simulink model "abl_M1_proposed"  (R2023b)
settings: Solver=ode45  StartTime=0.0  StopTime=80  MaxStep=1e-3  RelTol=5e-5
model workspace (MAT data in the model file):
  gpsid1 : Simulink.Signal (value not decoded)
  gpsid2 : Simulink.Signal (value not decoded)
  gpsid3 : Simulink.Signal (value not decoded)
  kkk1 : Simulink.Signal (value not decoded)
  kkk2 : Simulink.Signal (value not decoded)
  kkk3 : Simulink.Signal (value not decoded)
  psid = 0.5
undefined symbols (not defined in the file): A_raw1, A_raw2, beta1, beta2, p00, p_d_10, p_d_20, p_d_30, p_d_40, p_d_50, p_d_60, p_hat_p10, p_hat_p20, p_hat_p30, p_hat_p40, p_hat_p50, p_hat_p60, p_hat_v10, p_hat_v20, p_hat_v30, p_hat_v40, p_hat_v50, p_hat_v60, p_off_set1, p_off_set2, v00
(part 4 of 4)

== matlab function abl_M1_proposed/MATLAB Function1 ==
  settings: updateMethod=DISCRETE
  data: t input; dp_hat_i output; p0 input; v0 input; p_hat_all input; v_hat_all input; p_d_all input; id input; A_row input; beta input; p_offset input; dv_hat_i output; dp_d_i output
function [dp_hat_i, dv_hat_i, dp_d_i] = Follower_Model(t, p0, v0, p_hat_all, v_hat_all, p_d_all, id, A_row, beta, p_offset)
    % 输入说明:
    % t: 仿真时间 (Clock)
    % p0, v0: 领航者真实状态 (仅在beta_i > 0时起作用)
    % p_hat_all, v_hat_all, p_d_all: 所有跟随者的状态矩阵 (外部合并后传入)
    % id: 当前智能体编号
    % A_row: 当前智能体对其他人的邻接权重 (用于检测网络拓扑变化)
    % beta_i: 当前智能体是否能直接观测到领航者 (1或0)
    % p_offset: 期望与目标的相对编队位置偏置 (2x1 向量)

    % --- 仿真参数设定 ---
    kp_l = 0.5; 
    phi_p = 2.0; 
    Ta = 5.0;         % 规定观测器收敛时间
    Omega_bar = 4; 
    k1 = 0.1; 
    lambda = 1.0; 
    Tp = 10.0;      % 规定围住控制形成的时间
    d_avoid = 10;    % 避碰距离 d
    mu = 20;         % 避碰范围上限 mu

    % === 自动重启机制核心逻辑 ===
    % 使用 persistent 变量存储上一时刻的拓扑和最近一次的切换时间 tk
    persistent tk A_row_prev;
    
    if isempty(tk)
        tk = 0;
        A_row_prev = A_row;
    end
    
    % 检测到邻接权重矩阵发生改变，说明有智能体加入/退出，更新重启时刻 tk
    if any(A_row ~= A_row_prev)
        tk = t;
        A_row_prev = A_row;
    end
    
    % 计算自上次拓扑切换以来经过的“局部时间”
    t_local = t - tk; 
    % ===========================

    p_hat_i = p_hat_all(2*(id-1)+1:2*id);
    v_hat_i = v_hat_all(2*(id-1)+1:2*id);
    p_d_i = p_d_all(2*(id-1)+1:2*id);

    %% ---------------- A. 移动目标规定时间观测器 ----------------
    sum_p = zeros(size(p_hat_i));
    sum_v = zeros(size(v_hat_i));
    % 这里的循环处理完美契合“无标签”特性：不管是谁，只要 A_row(j)>0 就计算
    for j = 1:size(beta, 1)
        if A_row(id,j) > 0 && j ~= id
            sum_p = sum_p + A_row(id,j) * (p_hat_i - p_hat_all(2*(j-1)+1:2*j));
            sum_v = sum_v + A_row(id,j) * (v_hat_i - v_hat_all(2*(j-1)+1:2*j));
        end
    end
    
    eta_ip = sum_p + beta(id) * (p_hat_i - p0);
    eta_iv = sum_v + beta(id) * (v_hat_i - v0);

    % 观测器时变增益 kp (基于局部时间 t_local 重启)
    % 引入 -0.01 防止时间刚好等于 Ta 时分母为 0
    if t_local < Ta - 0.001 
        kp = kp_l + 1/(2*phi_p) + 2/(Ta - t_local);
    else
        kp = kp_l + 1/(2*phi_p);
    end

    sig_eta_iv = sign(eta_iv); 
    dp_hat_i = v_hat_i - kp * eta_ip;
    dv_hat_i = -kp * eta_iv - Omega_bar * sig_eta_iv;

    %% ---------------- B. 无标签目标围捕导航层 ----------------
    % 导航层时变增益 k (基于局部时间 t_local 重启)
    if t_local < Tp - 0.2
        k_gain = k1 + 0.01 + lambda/(Tp - t_local);
    else
        k_gain = k1 + 0.01;
    end

    p_tilde_d_i = p_d_i - p_hat_i - 0*p_offset(:,id); 
    m_gain = 100;
    sum_avoid = zeros(size(p_d_i));
    for j = 1:size(beta, 1)
        if A_row(id,j) > 0 && j ~= id
            p_d_ij = p_d_i - p_d_all(2*(j-1)+1:2*j);
            norm_p = norm(p_d_ij);
            
            if norm_p > d_avoid && norm_p <= mu
                alpha_val = 1/(norm_p - d_avoid) - 1/(mu - d_avoid);
            else
                alpha_val = 0; % 超出感知范围，或者发生了不可逆穿透，斥力置0防崩溃
            end
            
            if norm_p > 0
                % + 号表示顺着 p_d_ij 的方向把自己推开
                sum_avoid = sum_avoid + m_gain * alpha_val * (p_d_ij / norm_p);
            end
        end
    end
    p_d_ij = p_d_i - p_hat_i;
    norm_p = norm(p_d_ij);
            
    if norm_p > d_avoid && norm_p <= mu
        alpha_val = 1/(norm_p - d_avoid) - 1/(mu - d_avoid);
    else
        alpha_val = 0; % 超出感知范围，或者发生了不可逆穿透，斥力置0防崩溃
    end
    
    if norm_p > 0
        % + 号表示顺着 p_d_ij 的方向把自己推开
        sum_avoid = sum_avoid + m_gain * alpha_val * (p_d_ij / norm_p);
    end
    % v_d_i = 速度前馈 - 引力 + 斥力
    v_d_i = v_hat_i - k_gain *(p_tilde_d_i -sum_avoid);
    dp_d_i = v_d_i;
end

== matlab function abl_M1_proposed/Subsystem18/Subsystem/Guidence ==
  settings: updateMethod=DISCRETE
  data: t input; x input; y input; desire input; psi input; psid output; psi_e output; rhoe output; xd output; yd output
function [psid,psi_e,rhoe,xd,yd]  = desire(t,x,y,desire,psi)
xd = desire(1);yd = desire(4);
dxd = desire(2); dyd=desire(5);
xe =x-xd;
ye =y-yd;
 rhoe = sqrt((xe)^2+(ye)^2); 
 persistent kkk2 gpsid2
% if abs(rhoe)<1
    p = atan2(10000*ye+10*dyd,10000*xe+10*dxd);
    % u1 = 0.1*dxd+10*xe;
    % u2 = 0.1*dyd+10*ye;
    % z=u1+u2*i;
    % p=angle(z);
% else
%     p = atan2(ye,xe);
% end

if isempty(kkk2)
    kkk2=0;
    gpsid2=p;
end
if p*gpsid2<-0.7*pi^2 && p>0  %Change nearly in -pi and +pi
   kkk2=kkk2-1;
end
if p*gpsid2<-0.7*pi^2 && p<0  %Change nearly in -pi and +pi
   kkk2=kkk2+1;
end
gpsid2=p;
psid=p+2*kkk2*pi;
psi_e = psi-psid;
 
 

end

== matlab function abl_M1_proposed/Subsystem18/Subsystem1/MATLAB Function1 ==
  data: x1 input; dotx1 output; dotx2 output; x2 input; psid input
function [dotx1,dotx2] = desire(x1,x2,psid)
    R  = 1;
    dotx1 = x2;
    dotx2 = -2*R^2*(x1-psid)-R*x2;
end

== matlab function abl_M1_proposed/Subsystem18/Subsystem1/MATLAB Function2 ==
  data: x1 input; dotx1 output; dotx2 output; x2 input; psid input
function [dotx1,dotx2] = desire(x1,x2,psid)
    R  = 1;
    dotx1 = x2;
    dotx2 = -2*R^2*(x1-psid)-R*x2;
end

== matlab function abl_M1_proposed/USV8/MATLAB Function ==
  data: t input; tau_u input; x_dot output; y_dot output; psi_dot output; u_dot output; v_dot output; r_dot output; tau_r input; psi input; u input; v input; r input
function [x_dot, y_dot, psi_dot, u_dot, v_dot, r_dot] = dynamics(t,tau_u,tau_r,psi,u, v, r)
    m11=24.9;m22=33.8;m33=2.86;
    Du=12;Dv=17;Dr=0.5;
    % Kinematic equations
    x_dot = u * cos(psi) - v * sin(psi);
    y_dot = u * sin(psi) + v * cos(psi);    
    psi_dot = r;
    % Disturbence
    tau_wu = 0.50*sin(0.1*t);
    tau_wv = 0.50*cos(0.1*t); 
    tau_wr = 0.50*sin(0.2*t);
    % Dynamic equations
    u_dot = (m22 * v * r - Du * u + tau_u + tau_wu) / m11;
    v_dot = (-m11 * u * r - Dv * v + tau_wv) / m22;
    r_dot = ((m11 - m22) * u * v - Dr * r + tau_r + tau_wr) / m33;
    % 质量和惯性参数
   

end

== matlab function abl_M1_proposed/USV9/MATLAB Function ==
  data: t input; tau_u input; x_dot output; y_dot output; psi_dot output; u_dot output; v_dot output; r_dot output; tau_r input; psi input; u input; v input; r input
function [x_dot, y_dot, psi_dot, u_dot, v_dot, r_dot] = dynamics(t,tau_u,tau_r,psi,u, v, r)
    m11=24.9;m22=33.8;m33=2.86;
    Du=12;Dv=17;Dr=0.5;
    % Kinematic equations
    x_dot = u * cos(psi) - v * sin(psi);
    y_dot = u * sin(psi) + v * cos(psi);    
    psi_dot = r;
    % Disturbence
    tau_wu = 0.50*sin(0.1*t);
    tau_wv = 0.50*cos(0.1*t); 
    tau_wr = 0.50*sin(0.2*t);
    % Dynamic equations
    u_dot = (m22 * v * r - Du * u + tau_u + tau_wu) / m11;
    v_dot = (-m11 * u * r - Dv * v + tau_wv) / m22;
    r_dot = ((m11 - m22) * u * v - Dr * r + tau_r + tau_wr) / m33;
    % 质量和惯性参数
   

end
